simulink library "Sensors_Lib"  (R2016b)
settings: Solver=ode45  StartTime=0.0  StopTime=10.0  RelTol=1e-3  EnableMultiTasking=on
values from neighbouring files (symbols this model uses):
  AC =     [UAV_modelconfig.mat]
undefined symbols (not defined in the file or in its folder): sens
libraries: Sensors_Lib x31, OpenFlightUtilLib x7, simulink x2
settings Model: Creator=University of Minnesota  LastModifiedBy=rega0051
settings DataIOCC: LimitDataPoints=on  SaveFormat=Array  SignalLoggingSaveFormat=ModelDataLogs
settings OptimizationCC: ExpressionDepthLimit=2147483647  LifeSpan=inf  SimCompilerOptimization=on
settings DebuggingCC: UnderspecifiedInitializationDetection=Classic  MergeDetectMultiDrivingBlocksExec=none  SolverPrmCheckMsg=warning  FcnCallInpInsideContextMsg=warning  StateNameClashWarn=warning  StrictBusMsg=Warning  SFUnexpectedBacktrackingDiag=warning  SFNoUnconditionalDefaultTransitionDiag=warning  SFExecutionAtInitializationDiag=none
settings HardwareCC: ProdBitPerPointer=32  ProdBitPerSizeT=32  ProdBitPerPtrDiffT=32  ProdLargestAtomicFloat=None  ProdIntDivRoundTo=Undefined  ProdEndianess=Unspecified  ProdWordSize=32  ProdHWDeviceType=32-bit Generic
settings ModelReferenceCC: PropagateSignalLabelsOutOfModel=off
settings GRTTargetCC: TargetLangStandard=C89/C90 (ANSI)  GeneratePreprocessorConditionals=Disable all  CombineOutputUpdateFcns=off  GRTInterface=on
settings ConfigComp: CovMetricSettings=dw  CovHtmlReporting=on  CovSaveCumulativeToWorkspaceVar=on  CovSaveSingleToWorkspaceVar=on  CovExternalEMLEnable=off

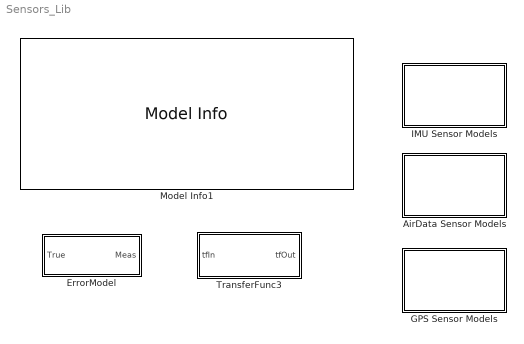
== system Sensors_Lib ==
  AirData Sensor Models : Subsystem
  ErrorModel : Subsystem  mask(Sensor Error Model - Scale, Bias, Noise){enable=sens.errEnable, scf=sens.sensScf, bias=sens.sensBias, sigma=sens.sensSigma, seed=sens.sensSeed, timestep=sens.timeSample_s}
      mask prompts: enable "Enable (on/off):"; scf "Scale Factor:"; sigma "Noise Sigma:"; seed "Noise Seed:"; timestep "Time Step (s):"
      mask help:
      | Apply a scale factor, add a bias and noise to a signal.
      |
      | - Enable (on/off): 1 = error on, 0 = error off.
      | - 'Scale Factor' : Scale factor applied to original signal (applied as a matrix multiplication).
      | - 'Bias'  : Constant offset bias (vectorized).
      | - 'Sigma' : Standard deviation of noise (vectorized).
      | - 'Noise Seed'  : Random number seed (vectorized).
      | - 'Time Step (s)': Time step for the noise generation.
      mask Display: disp('bias/scf/noise')
  GPS Sensor Models : Subsystem
  IMU Sensor Models : Subsystem
  Model Info1 : simulink/Model-Wide Utilities/Model Info  Frame=on  DisplayStringWithTags=|  HorizontalTextAlignment=Left  LeftAlignmentValue=0.02  SourceBlockDiagram=Sensors_Lib  TagMaxNumber=20
      | MODEL INFORMATION
      | Sensors Library (%<ModelName>)
      | 
      | University of Minnesota
      | Aerospace Engineering and Mechanics
      | Copyright 2017 Regents of the University of Minnesota. All rights reserved.
      | 
      | == Update Info ==
      | Last modified by %<LastModifiedBy> on %<LastModificationDate>
  TransferFunc3 : Subsystem  mask(Transfer Function (3)){tf_num=sens.gyroTF_num, tf_den=sens.gyroTF_den}
      mask prompts: tf_num "Transfer Function Numerator:"; tf_den "Transfer Function Denominator:"
      mask help: Applies a Transfer Function to a vector signal of length 3. The same transfer function is applied to each signal in the vector.
      settings: AttributesFormatString=%<tf_num> / %<tf_den>

== system Sensors_Lib/AirData Sensor Models ==
  AirData_Err : Subsystem  VariantControl=Variant1
  AirData_LocErr : Subsystem  VariantControl=VarAirData_LocErr
  AirData_LocTransErr : Subsystem  VariantControl=VarAirData_LocTransErr
  AirData_Pass : Subsystem  VariantControl=Variant1
  Body2PitotStatic : Subsystem

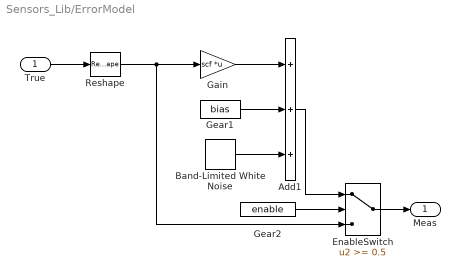
== system Sensors_Lib/ErrorModel ==
  True : Inport
  Add1 : Sum  Inputs=+++
  Band-Limited White Noise : simulink/Sources/Band-Limited White Noise  Cov=sigma  Ts=timestep  seed=seed
  EnableSwitch : Switch  Threshold=0.5  SaturateOnIntegerOverflow=on  InputSameDT=on
  Gain : Gain  Gain=scf  Multiplication=Matrix(K*u)
  Gear1 : Constant  Value=bias
  Gear2 : Constant  Value=enable
  Reshape : Reshape  OutputDimensionality=Column vector (2-D)
  Meas : Outport
  wires:
  Gain/1 -> Add1/1
  True/1 -> Reshape/1
  EnableSwitch/1 -> Meas/1
  Gear2/1 -> EnableSwitch/2
  Add1/1 -> EnableSwitch/1
  Gear1/1 -> Add1/2
  Band-Limited White Noise/1 -> Add1/3
  Reshape/1 -> Gain/1, EnableSwitch/3

== system Sensors_Lib/GPS Sensor Models ==
  GPS_Err : Subsystem  VariantControl=Variant1
  GPS_LocErr : Subsystem  VariantControl=Variant1
  GPS_LocTransErr : Subsystem  VariantControl=Variant1
  GPS_Pass : Subsystem  VariantControl=Variant1

== system Sensors_Lib/IMU Sensor Models ==
  Body2IMU : Subsystem
  IMU_Err : Subsystem  VariantControl=VarImu_Err
  IMU_LocErr : Subsystem  VariantControl=VarImu_LocErr
  IMU_LocTransErr : Subsystem  VariantControl=VarImu_LocTransErr
  IMU_Pass : Subsystem  VariantControl=VarIMU_Pass

== system Sensors_Lib/TransferFunc3 ==
  tfIn : Inport
  Demux : Demux  Outputs=3
  Mux : Mux  Inputs=3
  Transfer Fcn : TransferFcn  Numerator=tf_num  Denominator=tf_den
  Transfer Fcn1 : TransferFcn  Numerator=tf_num  Denominator=tf_den
  Transfer Fcn2 : TransferFcn  Numerator=tf_num  Denominator=tf_den
  tfOut : Outport
  wires:
  tfIn/1 -> Demux/1
  Mux/1 -> tfOut/1
  Demux/1 -> Transfer Fcn/1
  Demux/2 -> Transfer Fcn1/1
  Demux/3 -> Transfer Fcn2/1
  Transfer Fcn/1 -> Mux/1
  Transfer Fcn1/1 -> Mux/2
  Transfer Fcn2/1 -> Mux/3

== system Sensors_Lib/AirData Sensor Models/AirData_Err ==
  States : Inport
  Bus Creator : BusCreator  Inputs=3  OutDataTypeStr=Bus: AirData
      settings: InheritFromInputs=off
  Bus Selector : BusSelector  OutputSignals=AuxVar.qBar_Pa,EnvData.Pressure_kPa,EnvData.Temperature_K
  ErrorModel : Sensors_Lib/ErrorModel  enable=sens.errEnable  scf=sens.PdScf  bias=sens.PdBias  sigma=sens.PdSigma  seed=sens.PdSeed  timestep=sens.timeSample_s
  ErrorModel1 : Sensors_Lib/ErrorModel  enable=sens.errEnable  scf=sens.PsScf  bias=sens.PsBias  sigma=sens.PsSigma  seed=sens.PsSeed  timestep=sens.timeSample_s
  ErrorModel2 : Sensors_Lib/ErrorModel  enable=sens.errEnable  scf=sens.tempScf  bias=sens.tempBias  sigma=sens.tempSigma  seed=sens.tempSeed  timestep=sens.timeSample_s
  AirData : Outport
  wires:
  Bus Selector/3 -> ErrorModel2/1  "<Temperature_K>"
  States/1 -> Bus Selector/1
  ErrorModel2/1 -> Bus Creator/3  "temp_K"
  ErrorModel1/1 -> Bus Creator/2  "Ps_Pa"
  ErrorModel/1 -> Bus Creator/1  "Pd_Pa"
  Bus Creator/1 -> AirData/1  "AirData"
  Bus Selector/1 -> ErrorModel/1  "<qBar_Pa>"
  Bus Selector/2 -> ErrorModel1/1  "<Pressure_kPa>"

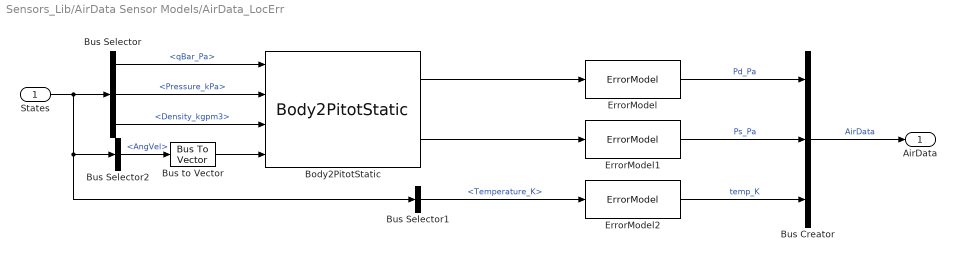
== system Sensors_Lib/AirData Sensor Models/AirData_LocErr ==
  States : Inport
  Body2PitotStatic : Sensors_Lib/AirData Sensor Models/Body2PitotStatic
  Bus Creator : BusCreator  Inputs=3  OutDataTypeStr=Bus: AirData
      settings: InheritFromInputs=off
  Bus Selector : BusSelector  OutputSignals=AuxVar.qBar_Pa,EnvData.Pressure_kPa,EnvData.Density_kgpm3
  Bus Selector1 : BusSelector  OutputSignals=EnvData.Temperature_K
  Bus Selector2 : BusSelector  OutputSignals=RigidStates.AngVel
  Bus to Vector : BusToVector
  ErrorModel : Sensors_Lib/ErrorModel  enable=sens.errEnable  scf=sens.PdScf  bias=sens.PdBias  sigma=sens.PdSigma  seed=sens.PdSeed  timestep=sens.timeSample_s
  ErrorModel1 : Sensors_Lib/ErrorModel  enable=sens.errEnable  scf=sens.PsScf  bias=sens.PsBias  sigma=sens.PsSigma  seed=sens.PsSeed  timestep=sens.timeSample_s
  ErrorModel2 : Sensors_Lib/ErrorModel  enable=sens.errEnable  scf=sens.tempScf  bias=sens.tempBias  sigma=sens.tempSigma  seed=sens.tempSeed  timestep=sens.timeSample_s
  AirData : Outport
  wires:
  Bus to Vector/1 -> Body2PitotStatic/4
  Bus Selector2/1 -> Bus to Vector/1  "<AngVel>"
  Bus Selector/3 -> Body2PitotStatic/3  "<Density_kgpm3>"
  Bus Selector1/1 -> ErrorModel2/1  "<Temperature_K>"
  Bus Creator/1 -> AirData/1  "AirData"
  ErrorModel/1 -> Bus Creator/1  "Pd_Pa"
  ErrorModel1/1 -> Bus Creator/2  "Ps_Pa"
  ErrorModel2/1 -> Bus Creator/3  "temp_K"
  States/1 -> Bus Selector/1, Bus Selector2/1, Bus Selector1/1
  Bus Selector/1 -> Body2PitotStatic/1  "<qBar_Pa>"
  Body2PitotStatic/1 -> ErrorModel/1
  Body2PitotStatic/2 -> ErrorModel1/1
  Bus Selector/2 -> Body2PitotStatic/2  "<Pressure_kPa>"

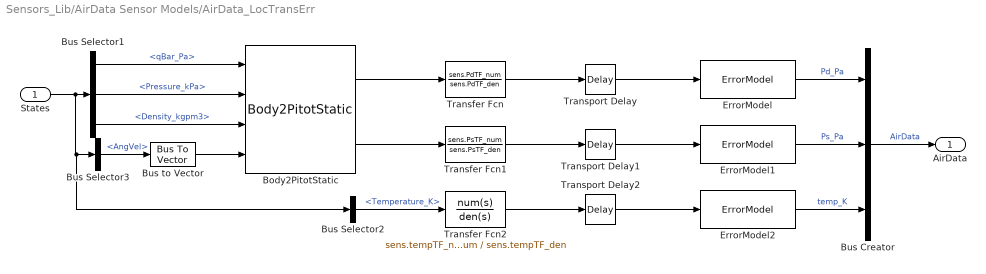
== system Sensors_Lib/AirData Sensor Models/AirData_LocTransErr ==
  States : Inport
  Body2PitotStatic : Sensors_Lib/AirData Sensor Models/Body2PitotStatic
  Bus Creator : BusCreator  Inputs=3  OutDataTypeStr=Bus: AirData
      settings: InheritFromInputs=off
  Bus Selector1 : BusSelector  OutputSignals=AuxVar.qBar_Pa,EnvData.Pressure_kPa,EnvData.Density_kgpm3
  Bus Selector2 : BusSelector  OutputSignals=EnvData.Temperature_K
  Bus Selector3 : BusSelector  OutputSignals=RigidStates.AngVel
  Bus to Vector : BusToVector
  ErrorModel : Sensors_Lib/ErrorModel  enable=sens.errEnable  scf=sens.PdScf  bias=sens.PdBias  sigma=sens.PdSigma  seed=sens.PdSeed  timestep=sens.timeSample_s
  ErrorModel1 : Sensors_Lib/ErrorModel  enable=sens.errEnable  scf=sens.PsScf  bias=sens.PsBias  sigma=sens.PsSigma  seed=sens.PsSeed  timestep=sens.timeSample_s
  ErrorModel2 : Sensors_Lib/ErrorModel  enable=sens.errEnable  scf=sens.tempScf  bias=sens.tempBias  sigma=sens.tempSigma  seed=sens.tempSeed  timestep=sens.timeSample_s
  Transfer Fcn : TransferFcn  Numerator=sens.PdTF_num  Denominator=sens.PdTF_den
      settings: AttributesFormatString=|
      | %<Numerator>
      | %<Denominator>
  Transfer Fcn1 : TransferFcn  Numerator=sens.PsTF_num  Denominator=sens.PsTF_den
      settings: AttributesFormatString=|
      | %<Numerator>
      | %<Denominator>
  Transfer Fcn2 : TransferFcn  Numerator=sens.tempTF_num  Denominator=sens.tempTF_den
      settings: AttributesFormatString=|
      | %<Numerator>
      | %<Denominator>
  Transport Delay : TransportDelay  DelayTime=sens.PdTimeDelay_s  TransDelayFeedthrough=on  PadeOrder=2
      settings: AttributesFormatString=%<DelayTime>
  Transport Delay1 : TransportDelay  DelayTime=sens.PdTimeDelay_s  TransDelayFeedthrough=on  PadeOrder=2
      settings: AttributesFormatString=%<DelayTime>
  Transport Delay2 : TransportDelay  DelayTime=sens.tempTimeDelay_s  TransDelayFeedthrough=on  PadeOrder=2
      settings: AttributesFormatString=%<DelayTime>
  AirData : Outport
  wires:
  Bus Creator/1 -> AirData/1  "AirData"
  ErrorModel/1 -> Bus Creator/1  "Pd_Pa"
  ErrorModel1/1 -> Bus Creator/2  "Ps_Pa"
  ErrorModel2/1 -> Bus Creator/3  "temp_K"
  Body2PitotStatic/1 -> Transfer Fcn/1
  Body2PitotStatic/2 -> Transfer Fcn1/1
  Transfer Fcn/1 -> Transport Delay/1
  Transfer Fcn1/1 -> Transport Delay1/1
  Transfer Fcn2/1 -> Transport Delay2/1
  Transport Delay/1 -> ErrorModel/1
  Transport Delay1/1 -> ErrorModel1/1
  Transport Delay2/1 -> ErrorModel2/1
  Bus Selector3/1 -> Bus to Vector/1  "<AngVel>"
  Bus Selector1/3 -> Body2PitotStatic/3  "<Density_kgpm3>"
  States/1 -> Bus Selector2/1, Bus Selector3/1, Bus Selector1/1
  Bus Selector1/1 -> Body2PitotStatic/1  "<qBar_Pa>"
  Bus Selector1/2 -> Body2PitotStatic/2  "<Pressure_kPa>"
  Bus Selector2/1 -> Transfer Fcn2/1  "<Temperature_K>"
  Bus to Vector/1 -> Body2PitotStatic/4

== system Sensors_Lib/AirData Sensor Models/AirData_Pass ==
  States : Inport
  Bus Creator : BusCreator  Inputs=3  OutDataTypeStr=Bus: AirData
      settings: InheritFromInputs=off
  Bus Selector : BusSelector  OutputSignals=AuxVar.qBar_Pa,EnvData.Pressure_kPa,EnvData.Temperature_K
  AirData : Outport
  wires:
  Bus Selector/2 -> Bus Creator/2  "<Pressure_kPa>"
  Bus Selector/1 -> Bus Creator/1  "<qBar_Pa>"
  Bus Creator/1 -> AirData/1  "AirData"
  States/1 -> Bus Selector/1
  Bus Selector/3 -> Bus Creator/3  "<Temperature_K>"

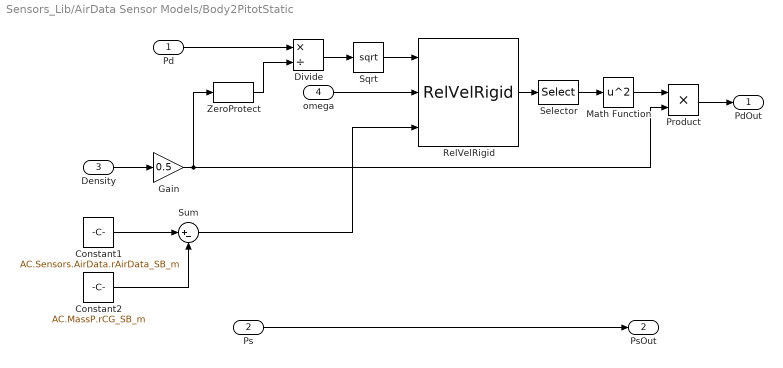
== system Sensors_Lib/AirData Sensor Models/Body2PitotStatic ==
  Pd : Inport
  Ps : Inport  Port=2
  Density : Inport  Port=3
  omega : Inport  Port=4
  Constant1 : Constant  Value=AC.Sensors.AirData.rAirData_SB_m
      settings: AttributesFormatString=%<Value>
  Constant2 : Constant  Value=AC.MassP.rCG_SB_m
      settings: AttributesFormatString=%<Value>
  Divide : Product  Inputs=*/
  Gain : Gain  Gain=0.5
  Math Function : Math  Operator=square  SaturateOnIntegerOverflow=on
  Product : Product
  RelVelRigid : OpenFlightUtilLib/Kinematics and Dynamics/RelVelRigid
  Selector : Selector  InputPortWidth=3  IndexOptions=Index vector (dialog)  Indices=1  OutputSizes=1
  Sqrt : Sqrt  SaturateOnIntegerOverflow=on
  Sum : Sum  Inputs=|+-
  ZeroProtect : OpenFlightUtilLib/Math/ZeroProtect  epsilon=eps
  PdOut : Outport
  PsOut : Outport  Port=2
  wires:
  ZeroProtect/1 -> Divide/2
  Selector/1 -> Math Function/1
  Sum/1 -> RelVelRigid/3
  Math Function/1 -> Product/1
  Gain/1 -> Product/2, ZeroProtect/1
  Density/1 -> Gain/1
  Product/1 -> PdOut/1
  omega/1 -> RelVelRigid/2
  Sqrt/1 -> RelVelRigid/1
  Divide/1 -> Sqrt/1
  Constant2/1 -> Sum/2
  Constant1/1 -> Sum/1
  Pd/1 -> Divide/1
  RelVelRigid/1 -> Selector/1
  Ps/1 -> PsOut/1

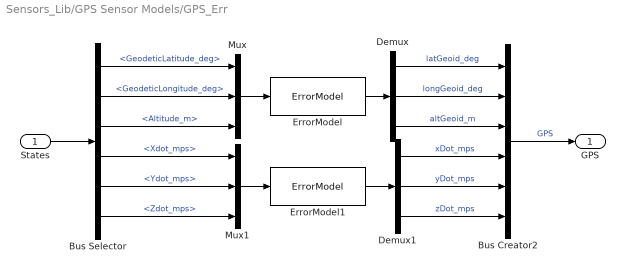
== system Sensors_Lib/GPS Sensor Models/GPS_Err ==
  States : Inport
  Bus Creator2 : BusCreator  Inputs=6  OutDataTypeStr=Bus: GPS
      settings: InheritFromInputs=off
  Bus Selector : BusSelector  OutputSignals=AuxVar.Nav.GeodeticLatitude_deg,AuxVar.Nav.GeodeticLongitude_deg,AuxVar.Nav.Altitude_m,AuxVar.V_e.Xdot_mps,AuxVar.V_e.Ydot_mps,AuxVar.V_e.Zdot_mps
  Demux : Demux  Outputs=3
  Demux1 : Demux  Outputs=3
  ErrorModel : Sensors_Lib/ErrorModel  enable=sens.errEnable  scf=sens.posScf  bias=sens.posBias  sigma=sens.posSigma  seed=sens.posSeed  timestep=sens.timeSample_s
  ErrorModel1 : Sensors_Lib/ErrorModel  enable=sens.errEnable  scf=sens.velScf  bias=sens.velBias  sigma=sens.velSigma  seed=sens.velSeed  timestep=sens.timeSample_s
  Mux : Mux  Inputs=3
  Mux1 : Mux  Inputs=3
  GPS : Outport
  wires:
  States/1 -> Bus Selector/1
  Demux/2 -> Bus Creator2/2  "longGeoid_deg"
  Demux/1 -> Bus Creator2/1  "latGeoid_deg"
  Demux/3 -> Bus Creator2/3  "altGeoid_m"
  Bus Selector/1 -> Mux/1  "<GeodeticLatitude_deg>"
  Bus Selector/2 -> Mux/2  "<GeodeticLongitude_deg>"
  Bus Selector/3 -> Mux/3  "<Altitude_m>"
  Bus Selector/6 -> Mux1/3  "<Zdot_mps>"
  Bus Selector/5 -> Mux1/2  "<Ydot_mps>"
  Bus Selector/4 -> Mux1/1  "<Xdot_mps>"
  Bus Creator2/1 -> GPS/1  "GPS"
  Mux/1 -> ErrorModel/1
  Demux1/1 -> Bus Creator2/4  "xDot_mps"
  Demux1/2 -> Bus Creator2/5  "yDot_mps"
  Demux1/3 -> Bus Creator2/6  "zDot_mps"
  ErrorModel/1 -> Demux/1
  Mux1/1 -> ErrorModel1/1
  ErrorModel1/1 -> Demux1/1

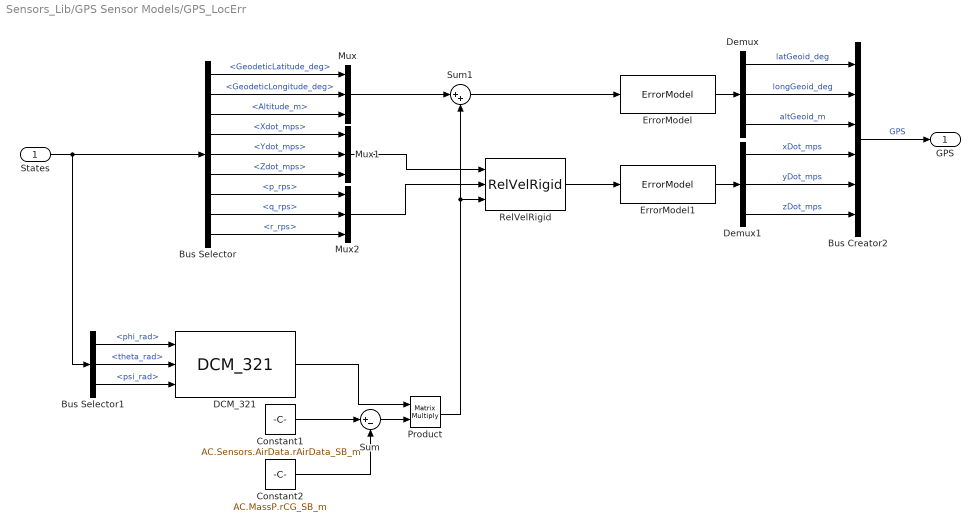
== system Sensors_Lib/GPS Sensor Models/GPS_LocErr ==
  States : Inport
  Bus Creator2 : BusCreator  Inputs=6  OutDataTypeStr=Bus: GPS
      settings: InheritFromInputs=off
  Bus Selector : BusSelector  OutputSignals=AuxVar.Nav.GeodeticLatitude_deg,AuxVar.Nav.GeodeticLongitude_deg,AuxVar.Nav.Altitude_m,AuxVar.V_e.Xdot_mps,AuxVar.V_e.Ydot_mps,AuxVar.V_e.Zdot_mps,RigidStates.AngVel.p_rps,RigidStates.AngVel.q_rps,RigidStates.AngVel.r_rps
  Bus Selector1 : BusSelector  OutputSignals=RigidStates.Euler.phi_rad,RigidStates.Euler.theta_rad,RigidStates.Euler.psi_rad
  Constant1 : Constant  Value=AC.Sensors.AirData.rAirData_SB_m
      settings: AttributesFormatString=%<Value>
  Constant2 : Constant  Value=AC.MassP.rCG_SB_m
      settings: AttributesFormatString=%<Value>
  DCM_321 : OpenFlightUtilLib/Transformations/DCM_321
  Demux : Demux  Outputs=3
  Demux1 : Demux  Outputs=3
  ErrorModel : Sensors_Lib/ErrorModel  enable=sens.errEnable  scf=sens.posScf  bias=sens.posBias  sigma=sens.posSigma  seed=sens.posSeed  timestep=sens.timeSample_s
  ErrorModel1 : Sensors_Lib/ErrorModel  enable=sens.errEnable  scf=sens.velScf  bias=sens.velBias  sigma=sens.velSigma  seed=sens.velSeed  timestep=sens.timeSample_s
  Mux : Mux  Inputs=3
  Mux1 : Mux  Inputs=3
  Mux2 : Mux  Inputs=3
  Product : Product  Multiplication=Matrix(*)
  RelVelRigid : OpenFlightUtilLib/Kinematics and Dynamics/RelVelRigid
  Sum : Sum  Inputs=|+-
  Sum1 : Sum  Inputs=|++
  GPS : Outport
  wires:
  States/1 -> Bus Selector1/1, Bus Selector/1
  Demux/2 -> Bus Creator2/2  "longGeoid_deg"
  Demux/1 -> Bus Creator2/1  "latGeoid_deg"
  Demux/3 -> Bus Creator2/3  "altGeoid_m"
  Bus Selector/1 -> Mux/1  "<GeodeticLatitude_deg>"
  Bus Selector/2 -> Mux/2  "<GeodeticLongitude_deg>"
  Bus Selector/3 -> Mux/3  "<Altitude_m>"
  Bus Selector/6 -> Mux1/3  "<Zdot_mps>"
  Bus Selector/5 -> Mux1/2  "<Ydot_mps>"
  Bus Selector/4 -> Mux1/1  "<Xdot_mps>"
  Bus Creator2/1 -> GPS/1  "GPS"
  Demux1/1 -> Bus Creator2/4  "xDot_mps"
  Demux1/2 -> Bus Creator2/5  "yDot_mps"
  Demux1/3 -> Bus Creator2/6  "zDot_mps"
  ErrorModel/1 -> Demux/1
  ErrorModel1/1 -> Demux1/1
  Constant1/1 -> Sum/1
  Constant2/1 -> Sum/2
  Sum/1 -> Product/2
  DCM_321/1 -> Product/1
  Product/1 -> Sum1/2, RelVelRigid/3
  Mux/1 -> Sum1/1
  Sum1/1 -> ErrorModel/1
  RelVelRigid/1 -> ErrorModel1/1
  Mux1/1 -> RelVelRigid/1
  Bus Selector1/1 -> DCM_321/1  "<phi_rad>"
  Bus Selector1/2 -> DCM_321/2  "<theta_rad>"
  Bus Selector1/3 -> DCM_321/3  "<psi_rad>"
  Mux2/1 -> RelVelRigid/2
  Bus Selector/8 -> Mux2/2  "<q_rps>"
  Bus Selector/7 -> Mux2/1  "<p_rps>"
  Bus Selector/9 -> Mux2/3  "<r_rps>"

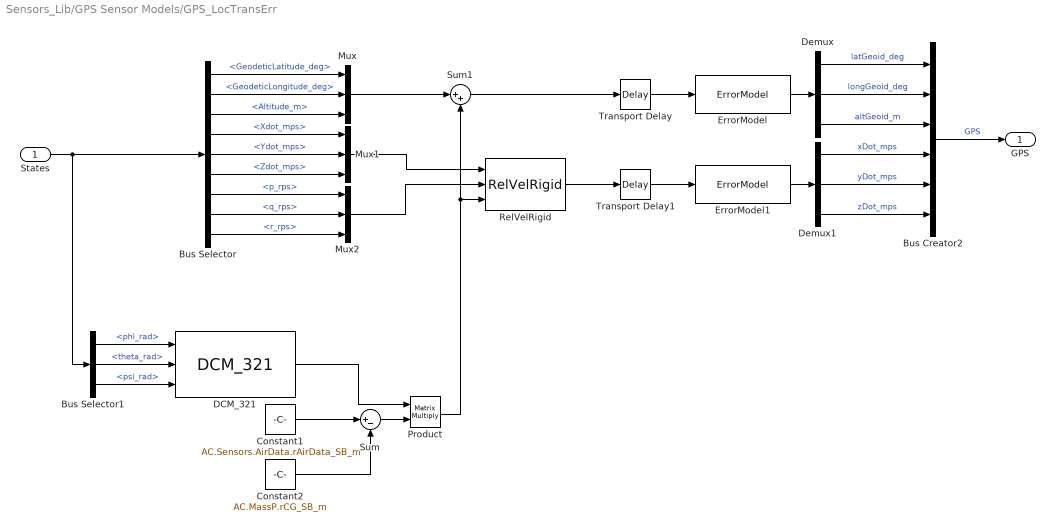
== system Sensors_Lib/GPS Sensor Models/GPS_LocTransErr ==
  States : Inport
  Bus Creator2 : BusCreator  Inputs=6  OutDataTypeStr=Bus: GPS
      settings: InheritFromInputs=off
  Bus Selector : BusSelector  OutputSignals=AuxVar.Nav.GeodeticLatitude_deg,AuxVar.Nav.GeodeticLongitude_deg,AuxVar.Nav.Altitude_m,AuxVar.V_e.Xdot_mps,AuxVar.V_e.Ydot_mps,AuxVar.V_e.Zdot_mps,RigidStates.AngVel.p_rps,RigidStates.AngVel.q_rps,RigidStates.AngVel.r_rps
  Bus Selector1 : BusSelector  OutputSignals=RigidStates.Euler.phi_rad,RigidStates.Euler.theta_rad,RigidStates.Euler.psi_rad
  Constant1 : Constant  Value=AC.Sensors.AirData.rAirData_SB_m
      settings: AttributesFormatString=%<Value>
  Constant2 : Constant  Value=AC.MassP.rCG_SB_m
      settings: AttributesFormatString=%<Value>
  DCM_321 : OpenFlightUtilLib/Transformations/DCM_321
  Demux : Demux  Outputs=3
  Demux1 : Demux  Outputs=3
  ErrorModel : Sensors_Lib/ErrorModel  enable=sens.errEnable  scf=sens.posScf  bias=sens.posBias  sigma=sens.posSigma  seed=sens.posSeed  timestep=sens.timeSample_s
  ErrorModel1 : Sensors_Lib/ErrorModel  enable=sens.errEnable  scf=sens.velScf  bias=sens.velBias  sigma=sens.velSigma  seed=sens.velSeed  timestep=sens.timeSample_s
  Mux : Mux  Inputs=3
  Mux1 : Mux  Inputs=3
  Mux2 : Mux  Inputs=3
  Product : Product  Multiplication=Matrix(*)
  RelVelRigid : OpenFlightUtilLib/Kinematics and Dynamics/RelVelRigid
  Sum : Sum  Inputs=|+-
  Sum1 : Sum  Inputs=|++
  Transport Delay : TransportDelay  DelayTime=sens.timeDelay_s  TransDelayFeedthrough=on  PadeOrder=2
      settings: AttributesFormatString=%<DelayTime>
  Transport Delay1 : TransportDelay  DelayTime=sens.timeDelay_s  TransDelayFeedthrough=on  PadeOrder=2
      settings: AttributesFormatString=%<DelayTime>
  GPS : Outport
  wires:
  Transport Delay1/1 -> ErrorModel1/1
  Transport Delay/1 -> ErrorModel/1
  Bus Selector/9 -> Mux2/3  "<r_rps>"
  Bus Selector/7 -> Mux2/1  "<p_rps>"
  Bus Selector/8 -> Mux2/2  "<q_rps>"
  Mux2/1 -> RelVelRigid/2
  Bus Selector1/3 -> DCM_321/3  "<psi_rad>"
  Bus Selector1/2 -> DCM_321/2  "<theta_rad>"
  Bus Selector1/1 -> DCM_321/1  "<phi_rad>"
  Mux1/1 -> RelVelRigid/1
  RelVelRigid/1 -> Transport Delay1/1
  Sum1/1 -> Transport Delay/1
  Mux/1 -> Sum1/1
  Product/1 -> RelVelRigid/3, Sum1/2
  DCM_321/1 -> Product/1
  Sum/1 -> Product/2
  Constant2/1 -> Sum/2
  Constant1/1 -> Sum/1
  ErrorModel1/1 -> Demux1/1
  ErrorModel/1 -> Demux/1
  Demux1/3 -> Bus Creator2/6  "zDot_mps"
  Demux1/2 -> Bus Creator2/5  "yDot_mps"
  Demux1/1 -> Bus Creator2/4  "xDot_mps"
  Bus Creator2/1 -> GPS/1  "GPS"
  Bus Selector/4 -> Mux1/1  "<Xdot_mps>"
  Bus Selector/5 -> Mux1/2  "<Ydot_mps>"
  Bus Selector/6 -> Mux1/3  "<Zdot_mps>"
  Bus Selector/3 -> Mux/3  "<Altitude_m>"
  Bus Selector/2 -> Mux/2  "<GeodeticLongitude_deg>"
  Bus Selector/1 -> Mux/1  "<GeodeticLatitude_deg>"
  Demux/3 -> Bus Creator2/3  "altGeoid_m"
  Demux/1 -> Bus Creator2/1  "latGeoid_deg"
  Demux/2 -> Bus Creator2/2  "longGeoid_deg"
  States/1 -> Bus Selector/1, Bus Selector1/1

== system Sensors_Lib/GPS Sensor Models/GPS_Pass ==
  States : Inport
  Bus Creator2 : BusCreator  Inputs=6  OutDataTypeStr=Bus: GPS
      settings: InheritFromInputs=off
  Bus Selector : BusSelector  OutputSignals=AuxVar.Nav.GeodeticLatitude_deg,AuxVar.Nav.GeodeticLongitude_deg,AuxVar.Nav.Altitude_m,AuxVar.V_e.Xdot_mps,AuxVar.V_e.Ydot_mps,AuxVar.V_e.Zdot_mps
  GPS : Outport
  wires:
  States/1 -> Bus Selector/1
  Bus Selector/1 -> Bus Creator2/1  "<GeodeticLatitude_deg>"
  Bus Selector/3 -> Bus Creator2/3  "<Altitude_m>"
  Bus Selector/2 -> Bus Creator2/2  "<GeodeticLongitude_deg>"
  Bus Selector/6 -> Bus Creator2/6  "<Zdot_mps>"
  Bus Selector/4 -> Bus Creator2/4  "<Xdot_mps>"
  Bus Creator2/1 -> GPS/1  "GPS"
  Bus Selector/5 -> Bus Creator2/5  "<Ydot_mps>"

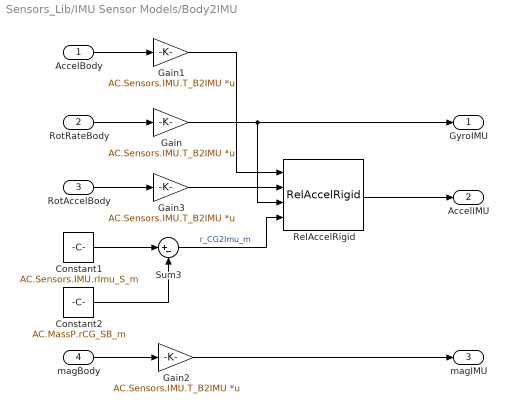
== system Sensors_Lib/IMU Sensor Models/Body2IMU ==
  AccelBody : Inport
  RotRateBody : Inport  Port=2
  RotAccelBody : Inport  Port=3
  magBody : Inport  Port=4
  Constant1 : Constant  Value=AC.Sensors.IMU.rImu_S_m
      settings: AttributesFormatString=%<Value>
  Constant2 : Constant  Value=AC.MassP.rCG_SB_m
      settings: AttributesFormatString=%<Value>
  Gain{,1..3} (4 alike) : Gain  Gain=AC.Sensors.IMU.T_B2IMU  Multiplication=Matrix(K*u)
      settings: AttributesFormatString=%<Gain>
  RelAccelRigid : OpenFlightUtilLib/Kinematics and Dynamics/RelAccelRigid
  Sum3 : Sum  Inputs=|+-  SaturateOnIntegerOverflow=on
  GyroIMU : Outport
  AccelIMU : Outport  Port=2
  magIMU : Outport  Port=3
  wires:
  RotRateBody/1 -> Gain/1
  AccelBody/1 -> Gain1/1
  Constant2/1 -> Sum3/2
  Constant1/1 -> Sum3/1
  Sum3/1 -> RelAccelRigid/4  "r_CG2Imu_m"
  RelAccelRigid/1 -> AccelIMU/1
  Gain2/1 -> magIMU/1
  Gain1/1 -> RelAccelRigid/1
  Gain/1 -> GyroIMU/1, RelAccelRigid/3
  RotAccelBody/1 -> Gain3/1
  Gain3/1 -> RelAccelRigid/2
  magBody/1 -> Gain2/1

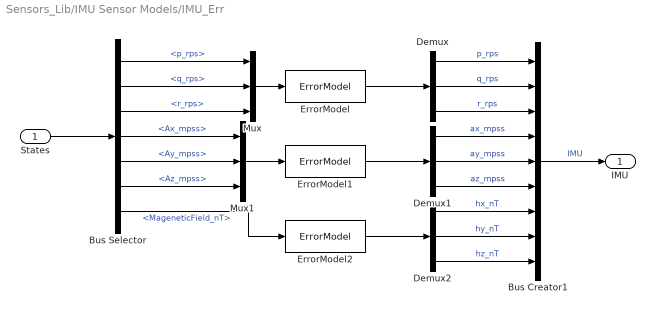
== system Sensors_Lib/IMU Sensor Models/IMU_Err ==
  States : Inport
  Bus Creator1 : BusCreator  Inputs=9  OutDataTypeStr=Bus: IMU
      settings: InheritFromInputs=off
  Bus Selector : BusSelector  OutputSignals=RigidStates.AngVel.p_rps,RigidStates.AngVel.q_rps,RigidStates.AngVel.r_rps,RigidStates.Accels.Ax_mpss,RigidStates.Accels.Ay_mpss,RigidStates.Accels.Az_mpss,EnvData.MageneticField_nT
  Demux : Demux  Outputs=3
  Demux1 : Demux  Outputs=3
  Demux2 : Demux  Outputs=3
  ErrorModel : Sensors_Lib/ErrorModel  enable=sens.errEnable  scf=sens.gyroScf  bias=sens.gyroBias  sigma=sens.gyroSigma  seed=sens.gyroSeed  timestep=sens.timeSample_s
  ErrorModel1 : Sensors_Lib/ErrorModel  enable=sens.errEnable  scf=sens.accelScf  bias=sens.accelBias  sigma=sens.accelSigma  seed=sens.accelSeed  timestep=sens.timeSample_s
  ErrorModel2 : Sensors_Lib/ErrorModel  enable=sens.errEnable  scf=sens.magScf  bias=sens.magBias  sigma=sens.magSigma  seed=sens.magSeed  timestep=sens.timeSample_s
  Mux : Mux  Inputs=3
  Mux1 : Mux  Inputs=3
  IMU : Outport
  wires:
  Demux2/3 -> Bus Creator1/9  "hz_nT"
  Demux2/2 -> Bus Creator1/8  "hy_nT"
  Demux2/1 -> Bus Creator1/7  "hx_nT"
  ErrorModel2/1 -> Demux2/1
  Bus Selector/7 -> ErrorModel2/1  "<MageneticField_nT>"
  ErrorModel1/1 -> Demux1/1
  Mux1/1 -> ErrorModel1/1
  Demux/3 -> Bus Creator1/3  "r_rps"
  Demux/2 -> Bus Creator1/2  "q_rps"
  Mux/1 -> ErrorModel/1
  ErrorModel/1 -> Demux/1
  Demux1/3 -> Bus Creator1/6  "az_mpss"
  Demux1/2 -> Bus Creator1/5  "ay_mpss"
  Demux1/1 -> Bus Creator1/4  "ax_mpss"
  Demux/1 -> Bus Creator1/1  "p_rps"
  Bus Creator1/1 -> IMU/1  "IMU"
  Bus Selector/6 -> Mux1/3  "<Az_mpss>"
  Bus Selector/5 -> Mux1/2  "<Ay_mpss>"
  Bus Selector/4 -> Mux1/1  "<Ax_mpss>"
  Bus Selector/3 -> Mux/3  "<r_rps>"
  Bus Selector/2 -> Mux/2  "<q_rps>"
  Bus Selector/1 -> Mux/1  "<p_rps>"
  States/1 -> Bus Selector/1

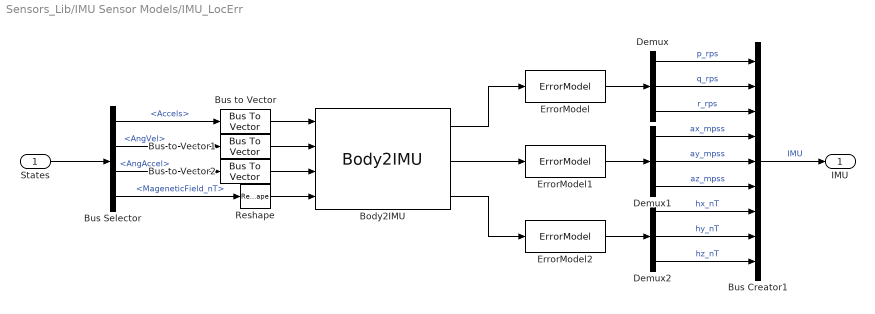
== system Sensors_Lib/IMU Sensor Models/IMU_LocErr ==
  States : Inport
  Body2IMU : Sensors_Lib/IMU Sensor Models/Body2IMU
  Bus Creator1 : BusCreator  Inputs=9  OutDataTypeStr=Bus: IMU
      settings: InheritFromInputs=off
  Bus Selector : BusSelector  OutputSignals=RigidStates.Accels,RigidStates.AngVel,RigidStates.AngAccel,EnvData.MageneticField_nT
  Bus to Vector : BusToVector
  Bus to Vector1 : BusToVector
  Bus to Vector2 : BusToVector
  Demux : Demux  Outputs=3
  Demux1 : Demux  Outputs=3
  Demux2 : Demux  Outputs=3
  ErrorModel : Sensors_Lib/ErrorModel  enable=sens.errEnable  scf=sens.gyroScf  bias=sens.gyroBias  sigma=sens.gyroSigma  seed=sens.gyroSeed  timestep=sens.timeSample_s
  ErrorModel1 : Sensors_Lib/ErrorModel  enable=sens.errEnable  scf=sens.accelScf  bias=sens.accelBias  sigma=sens.accelSigma  seed=sens.accelSeed  timestep=sens.timeSample_s
  ErrorModel2 : Sensors_Lib/ErrorModel  enable=sens.errEnable  scf=sens.magScf  bias=sens.magBias  sigma=sens.magSigma  seed=sens.magSeed  timestep=sens.timeSample_s
  Reshape : Reshape  OutputDimensionality=Column vector (2-D)
  IMU : Outport
  wires:
  States/1 -> Bus Selector/1
  Bus Creator1/1 -> IMU/1  "IMU"
  Demux/1 -> Bus Creator1/1  "p_rps"
  Demux1/1 -> Bus Creator1/4  "ax_mpss"
  Demux1/2 -> Bus Creator1/5  "ay_mpss"
  Demux1/3 -> Bus Creator1/6  "az_mpss"
  Demux/2 -> Bus Creator1/2  "q_rps"
  Demux/3 -> Bus Creator1/3  "r_rps"
  Demux2/1 -> Bus Creator1/7  "hx_nT"
  Demux2/2 -> Bus Creator1/8  "hy_nT"
  Demux2/3 -> Bus Creator1/9  "hz_nT"
  ErrorModel/1 -> Demux/1
  ErrorModel1/1 -> Demux1/1
  ErrorModel2/1 -> Demux2/1
  Bus Selector/4 -> Reshape/1  "<MageneticField_nT>"
  Body2IMU/1 -> ErrorModel/1
  Body2IMU/2 -> ErrorModel1/1
  Body2IMU/3 -> ErrorModel2/1
  Reshape/1 -> Body2IMU/4
  Bus to Vector/1 -> Body2IMU/1
  Bus to Vector1/1 -> Body2IMU/2
  Bus to Vector2/1 -> Body2IMU/3
  Bus Selector/1 -> Bus to Vector/1  "<Accels>"
  Bus Selector/2 -> Bus to Vector1/1  "<AngVel>"
  Bus Selector/3 -> Bus to Vector2/1  "<AngAccel>"

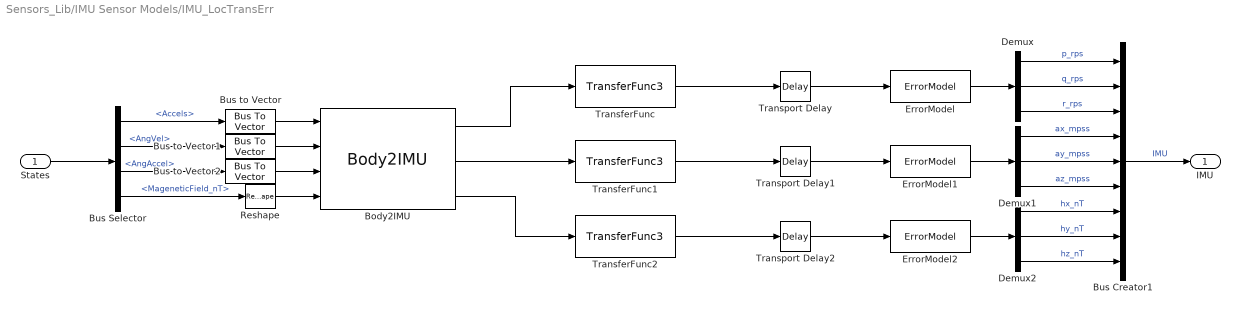
== system Sensors_Lib/IMU Sensor Models/IMU_LocTransErr ==
  States : Inport
  Body2IMU : Sensors_Lib/IMU Sensor Models/Body2IMU
  Bus Creator1 : BusCreator  Inputs=9  OutDataTypeStr=Bus: IMU
      settings: InheritFromInputs=off
  Bus Selector : BusSelector  OutputSignals=RigidStates.Accels,RigidStates.AngVel,RigidStates.AngAccel,EnvData.MageneticField_nT
  Bus to Vector : BusToVector
  Bus to Vector1 : BusToVector
  Bus to Vector2 : BusToVector
  Demux : Demux  Outputs=3
  Demux1 : Demux  Outputs=3
  Demux2 : Demux  Outputs=3
  ErrorModel : Sensors_Lib/ErrorModel  enable=sens.errEnable  scf=sens.gyroScf  bias=sens.gyroBias  sigma=sens.gyroSigma  seed=sens.gyroSeed  timestep=sens.timeSample_s
  ErrorModel1 : Sensors_Lib/ErrorModel  enable=sens.errEnable  scf=sens.accelScf  bias=sens.accelBias  sigma=sens.accelSigma  seed=sens.accelSeed  timestep=sens.timeSample_s
  ErrorModel2 : Sensors_Lib/ErrorModel  enable=sens.errEnable  scf=sens.magScf  bias=sens.magBias  sigma=sens.magSigma  seed=sens.magSeed  timestep=sens.timeSample_s
  Reshape : Reshape  OutputDimensionality=Column vector (2-D)
  TransferFunc : Sensors_Lib/TransferFunc3  tf_num=sens.gyroTF_num  tf_den=sens.gyroTF_den
      settings: AttributesFormatString=%<tf_num> / %<tf_den>
  TransferFunc1 : Sensors_Lib/TransferFunc3  tf_num=sens.accelTF_num  tf_den=sens.accelTF_den
      settings: AttributesFormatString=%<tf_num> / %<tf_den>
  TransferFunc2 : Sensors_Lib/TransferFunc3  tf_num=sens.magTF_num  tf_den=sens.magTF_den
      settings: AttributesFormatString=%<tf_num> / %<tf_den>
  Transport Delay : TransportDelay  DelayTime=sens.timeDelay_s  TransDelayFeedthrough=on  PadeOrder=2
      settings: AttributesFormatString=%<DelayTime>
  Transport Delay1 : TransportDelay  DelayTime=sens.timeDelay_s  TransDelayFeedthrough=on  PadeOrder=2
      settings: AttributesFormatString=%<DelayTime>
  Transport Delay2 : TransportDelay  DelayTime=sens.timeDelay_s  TransDelayFeedthrough=on  PadeOrder=2
      settings: AttributesFormatString=%<DelayTime>
  IMU : Outport
  wires:
  Bus Creator1/1 -> IMU/1  "IMU"
  Demux/1 -> Bus Creator1/1  "p_rps"
  Demux1/1 -> Bus Creator1/4  "ax_mpss"
  Demux1/2 -> Bus Creator1/5  "ay_mpss"
  Demux1/3 -> Bus Creator1/6  "az_mpss"
  Demux/2 -> Bus Creator1/2  "q_rps"
  Demux/3 -> Bus Creator1/3  "r_rps"
  Demux2/1 -> Bus Creator1/7  "hx_nT"
  Demux2/2 -> Bus Creator1/8  "hy_nT"
  Demux2/3 -> Bus Creator1/9  "hz_nT"
  ErrorModel/1 -> Demux/1
  ErrorModel1/1 -> Demux1/1
  ErrorModel2/1 -> Demux2/1
  Body2IMU/1 -> TransferFunc/1
  TransferFunc/1 -> Transport Delay/1
  Body2IMU/2 -> TransferFunc1/1
  Body2IMU/3 -> TransferFunc2/1
  TransferFunc1/1 -> Transport Delay1/1
  TransferFunc2/1 -> Transport Delay2/1
  Transport Delay/1 -> ErrorModel/1
  Transport Delay1/1 -> ErrorModel1/1
  Transport Delay2/1 -> ErrorModel2/1
  States/1 -> Bus Selector/1
  Bus Selector/4 -> Reshape/1  "<MageneticField_nT>"
  Reshape/1 -> Body2IMU/4
  Bus to Vector/1 -> Body2IMU/1
  Bus to Vector1/1 -> Body2IMU/2
  Bus to Vector2/1 -> Body2IMU/3
  Bus Selector/1 -> Bus to Vector/1  "<Accels>"
  Bus Selector/2 -> Bus to Vector1/1  "<AngVel>"
  Bus Selector/3 -> Bus to Vector2/1  "<AngAccel>"

== system Sensors_Lib/IMU Sensor Models/IMU_Pass ==
  note: IMU Passthrough Model
  States : Inport
  Bus Creator1 : BusCreator  Inputs=9  OutDataTypeStr=Bus: IMU
      settings: InheritFromInputs=off
  Bus Selector : BusSelector  OutputSignals=RigidStates.AngVel.p_rps,RigidStates.AngVel.q_rps,RigidStates.AngVel.r_rps,RigidStates.Accels.Ax_mpss,RigidStates.Accels.Ay_mpss,RigidStates.Accels.Az_mpss,EnvData.MageneticField_nT
  Demux3 : Demux  Outputs=3
  IMU : Outport
  wires:
  Demux3/3 -> Bus Creator1/9  "hz_nT"
  Demux3/2 -> Bus Creator1/8  "hy_nT"
  Demux3/1 -> Bus Creator1/7  "hx_nT"
  Bus Selector/7 -> Demux3/1  "<MageneticField_nT>"
  Bus Selector/5 -> Bus Creator1/5  "<Ay_mpss>"
  Bus Creator1/1 -> IMU/1  "IMU"
  Bus Selector/4 -> Bus Creator1/4  "<Ax_mpss>"
  Bus Selector/3 -> Bus Creator1/3  "<r_rps>"
  Bus Selector/2 -> Bus Creator1/2  "<q_rps>"
  Bus Selector/1 -> Bus Creator1/1  "<p_rps>"
  States/1 -> Bus Selector/1
  Bus Selector/6 -> Bus Creator1/6  "<Az_mpss>"
